simulink model "untitled"  (R2024a)
settings: Solver=VariableStepAuto  StartTime=0.0  StopTime=10.0  RelTol=1e-3
libraries: dspfdesign x1
settings Model: Creator=黄家睿  LastModifiedBy=黄家睿

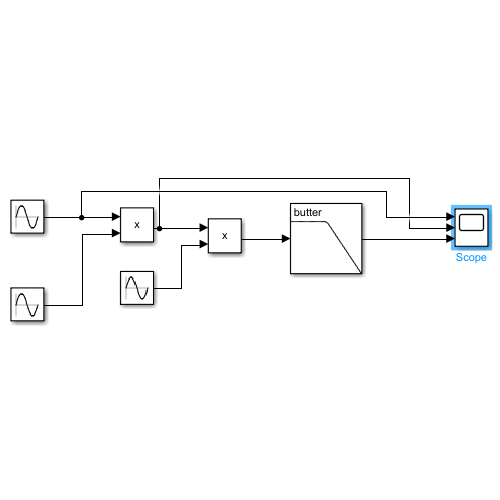
[thumbnail: Simulink's stored preview of the top-level diagram]
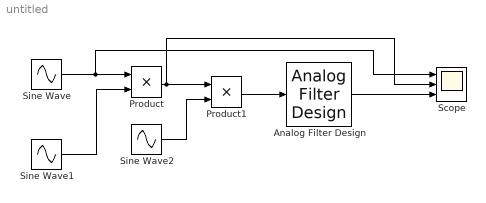
== system untitled ==
  Analog Filter Design : dspfdesign/Analog Filter Design  method=Butterworth  filttype=Lowpass  N=8  Wlo=6  Whi=80  Rp=2  Rs=40
  Product : Product
  Product1 : Product
  Scope : Scope  NumInputPorts=3
  Sine Wave : Sin  Frequency=5  SampleTime=0
  Sine Wave1 : Sin  Frequency=40  SampleTime=0
  Sine Wave2 : Sin  Frequency=40  SampleTime=0
  wires:
  Analog Filter Design/1 -> Scope/3
  Sine Wave/1 -> Scope/1, Product/1
  Sine Wave1/1 -> Product/2
  Sine Wave2/1 -> Product1/2
  Product1/1 -> Analog Filter Design/1
  Product/1 -> Scope/2, Product1/1
